simulink model "a6nl_sw_modelworkspace"  (R2020b)
settings: Solver=ode45  StartTime=0.0  StopTime=10.0  MaxStep=0.01  RelTol=1e-3  EnableMultiTasking=on
settings Model: Creator=Reichl  LastModifiedBy=jakob
settings DataIOCC: LimitDataPoints=on  SaveFormat=Array  SignalLoggingSaveFormat=ModelDataLogs  ReturnWorkspaceOutputs=off
settings OptimizationCC: ExpressionDepthLimit=2147483647  LifeSpan=inf
settings DebuggingCC: UnderspecifiedInitializationDetection=Classic  MergeDetectMultiDrivingBlocksExec=none  SolverPrmCheckMsg=warning  FcnCallInpInsideContextMsg=warning  StateNameClashWarn=warning  SFUnexpectedBacktrackingDiag=warning  SFNoUnconditionalDefaultTransitionDiag=warning  SFExecutionAtInitializationDiag=none  ArithmeticOperatorsInVariantConditions=warning
settings HardwareCC: ProdBitPerPointer=32  ProdBitPerSizeT=32  ProdBitPerPtrDiffT=32  ProdLargestAtomicFloat=None  ProdIntDivRoundTo=Undefined  ProdEndianess=Unspecified  ProdWordSize=32  ProdHWDeviceType=32-bit Generic
settings ModelReferenceCC: PropagateSignalLabelsOutOfModel=off
settings SFSimCC: SimUseLocalCustomCode=off  CustomCodeUndefinedFunction=UseInterfaceOnly
settings RTWCC: RTWUseLocalCustomCode=off
settings CodeAppCC: StateflowObjectComments=on
settings GRTTargetCC: TargetLangStandard=C89/C90 (ANSI)  CombineOutputUpdateFcns=off  GRTInterface=on
settings ConfigComp: CovMetricSettings=dw  CovSaveCumulativeToWorkspaceVar=on  CovSaveSingleToWorkspaceVar=on  CovExternalEMLEnable=off  CovSFcnEnable=off

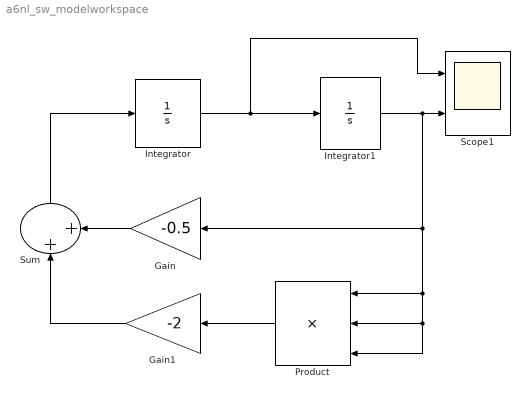
== system a6nl_sw_modelworkspace ==
  Gain : Gain  Gain=-0.5
  Gain1 : Gain  Gain=-2
  Integrator : Integrator
  Integrator1 : Integrator  InitialCondition=3
  Product : Product  Inputs=***  RndMeth=Zero
  Scope1 : Scope  NumInputPorts=2
  Sum : Sum  Inputs=|++
  wires:
  Integrator/1 -> Integrator1/1, Scope1/1
  Integrator1/1 -> Scope1/2, Product/3, Product/2, Product/1, Gain/1
  Gain/1 -> Sum/2
  Product/1 -> Gain1/1
  Gain1/1 -> Sum/1
  Sum/1 -> Integrator/1
